simulink model "TEMs_CV_I1"  (R2015a)
settings: Solver=ode3  StartTime=0.0  StopTime=1335  FixedStep=1  RelTol=5e-3
values from neighbouring files (symbols this model uses):
  B = 0.213*0.1143/2    (= 0.01217295)    [P_2CV_temNRTC_I.m]
  r_int = 0.18812    [P_2CV_temNRTC_I.m]
libraries: LU_TEG x4
settings Model: Creator=lansong7  LastModifiedBy=lansong7

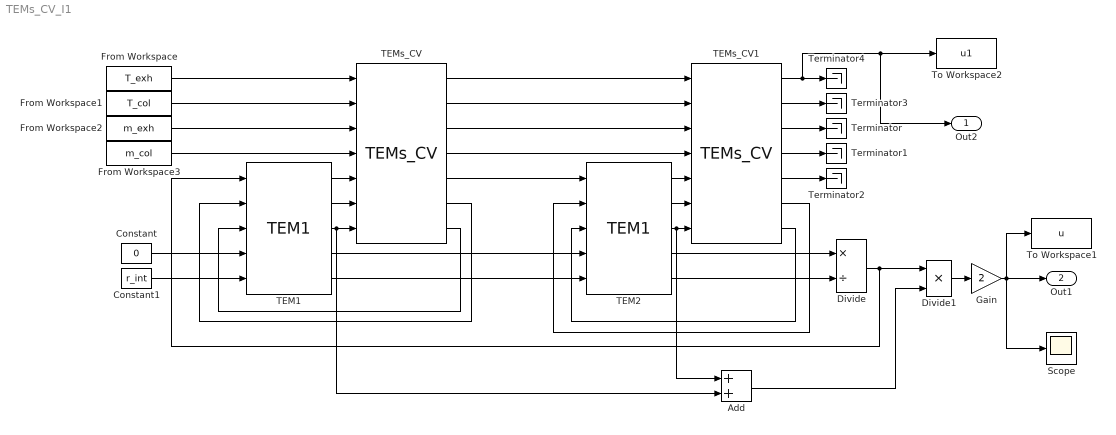
== system TEMs_CV_I1 ==
  Add : Sum
  Constant : Constant  Value=0
  Constant1 : Constant  Value=r_int
  Divide : Product  Inputs=*/
  Divide1 : Product  Inputs=**
  From Workspace : FromWorkspace  VariableName=T_exh  SampleTime=0
  From Workspace1 : FromWorkspace  VariableName=T_col  SampleTime=0
  From Workspace2 : FromWorkspace  VariableName=m_exh  SampleTime=0
  From Workspace3 : FromWorkspace  VariableName=m_col  SampleTime=0
  Gain : Gain  Gain=2
  Scope : Scope
  TEM1 : LU_TEG/TEM1  l=l  l_cw=l_cw  f=f  a=a  n=n  Tune_tr=Tune_tr  Tune_er=Tune_er  ct1=ct1  ct2=ct2  Parameter10=M
  TEM2 : LU_TEG/TEM1  l=l  l_cw=l_cw  f=f  a=a  n=n  Tune_tr=Tune_tr  Tune_er=Tune_er  ct1=ct1  ct2=ct2  Parameter10=M
  TEMs_CV : LU_TEG/TEMs_CV  B=B  a=a  side=side  l=l  l_cw=l_cw  M=M  M_hxr=M_hxr  M_ap=M_ap  C_hxr=C_hxr  C_ap=C_ap  l_hxr=l_hxr  b_hxr=b_hxr  a_hxr=a_hxr  Nf_hxr=Nf_hxr  tf_hxr=tf_hxr  M_cxr=M_cxr  C_cxr=C_cxr  Di_cxr=Di_cxr  T_hint=T_hint  T_cint=T_cint  ca1=ca1  ca2=ca2  ca3=ca3  cb1=cb1  cb2=cb2  cb3=cb3
  TEMs_CV1 : LU_TEG/TEMs_CV  B=B  a=a  side=side  l=l  l_cw=l_cw  M=M  M_hxr=M_hxr  M_ap=M_ap  C_hxr=C_hxr  C_ap=C_ap  l_hxr=l_hxr  b_hxr=b_hxr  a_hxr=a_hxr  Nf_hxr=Nf_hxr  tf_hxr=tf_hxr  M_cxr=M_cxr  C_cxr=C_cxr  Di_cxr=Di_cxr  T_hint=T_hint  T_cint=T_cint  ca1=ca1  ca2=ca2  ca3=ca3  cb1=cb1  cb2=cb2  cb3=cb3
  Terminator{,1..4} (5 alike) : Terminator
  To Workspace1 : ToWorkspace  VariableName=u  SaveFormat=Structure With Time  SampleTime=-1
  To Workspace2 : ToWorkspace  VariableName=u1  SaveFormat=Structure With Time  SampleTime=-1
  Out2 : Outport
  Out1 : Outport  Port=2
  wires:
  From Workspace2/1 -> TEMs_CV/3
  TEMs_CV/4 -> TEMs_CV1/4
  TEMs_CV/3 -> TEMs_CV1/3
  TEMs_CV/2 -> TEMs_CV1/2
  TEMs_CV/1 -> TEMs_CV1/1
  TEMs_CV1/3 -> Terminator/1
  TEMs_CV1/4 -> Terminator1/1
  TEMs_CV1/5 -> Terminator2/1
  TEMs_CV1/2 -> Terminator3/1
  TEMs_CV1/1 -> Out2/1, To Workspace2/1, Terminator4/1
  From Workspace1/1 -> TEMs_CV/2
  From Workspace3/1 -> TEMs_CV/4
  From Workspace/1 -> TEMs_CV/1
  Add/1 -> Divide1/2
  TEM1/1 -> TEMs_CV/5
  TEM1/2 -> TEMs_CV/6
  TEM1/3 -> Add/2, TEMs_CV/7
  TEM2/1 -> TEMs_CV1/5
  TEM2/2 -> TEMs_CV1/6
  TEM2/3 -> Add/1, TEMs_CV1/7
  Divide/1 -> TEM1/1, Divide1/1
  TEMs_CV/5 -> TEM2/1
  TEMs_CV/6 -> TEM1/2
  TEMs_CV/7 -> TEM1/3
  TEMs_CV1/7 -> TEM2/3
  TEMs_CV1/6 -> TEM2/2
  TEM1/5 -> TEM2/5
  TEM1/4 -> TEM2/4
  TEM2/4 -> Divide/1
  TEM2/5 -> Divide/2
  Constant1/1 -> TEM1/5
  Constant/1 -> TEM1/4
  Divide1/1 -> Gain/1
  Gain/1 -> To Workspace1/1, Scope/1, Out1/1
